simulink model "model"  (Simulink 7.5)
settings: Solver=ode45  StartTime=0.0  StopTime=500.0  RelTol=1e-3
settings Model: Creator=168092  LastModifiedBy=TC

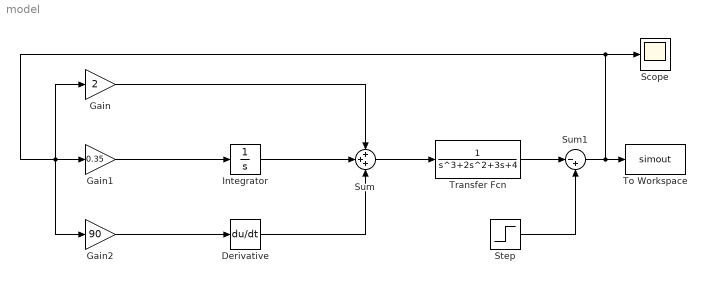
== system model ==
  Derivative : Derivative
  Gain : Gain  Gain=2  ParameterDataType=fixdt(1, 16)  ParameterScaling=2^0  OutDataType=fixdt(1, 16)  OutScaling=2^0
  Gain1 : Gain  Gain=0.35  ParameterDataType=fixdt(1, 16)  ParameterScaling=2^0  OutDataType=fixdt(1, 16)  OutScaling=2^0
  Gain2 : Gain  Gain=90  ParameterDataType=fixdt(1, 16)  ParameterScaling=2^0  OutDataType=fixdt(1, 16)  OutScaling=2^0
  Integrator : Integrator
  Scope : Scope
  Step : Step  SampleTime=0
  Sum : Sum  Inputs=+++  OutDataType=fixdt(1, 16)  OutScaling=2^0
  Sum1 : Sum  Inputs=|-+  OutDataType=fixdt(1, 16)  OutScaling=2^0
  To Workspace : ToWorkspace  VariableName=simout  SampleTime=-1  SaveFormat=Structure
  Transfer Fcn : TransferFcn  Denominator=[1 2 3 4]
  wires:
  Sum/1 -> Transfer Fcn/1
  Step/1 -> Sum1/2
  Transfer Fcn/1 -> Sum1/1
  Sum1/1 -> Scope/1, Gain/1, Gain2/1, Gain1/1, To Workspace/1
  Integrator/1 -> Sum/2
  Derivative/1 -> Sum/3
  Gain/1 -> Sum/1
  Gain2/1 -> Derivative/1
  Gain1/1 -> Integrator/1
